simulink model "motor_modelo_prelab"  (R2017b)
settings: Solver=FixedStepAuto  StartTime=0.0  StopTime=150  FixedStep=1/fs  RelTol=1e-3
values from neighbouring files (symbols this model uses):
  den_c = denc    [lab3.m]
  den_filtro = den2    [lab3.m]
  den_motor = den1    [lab3.m]
  fs = 100    [lab3.m]    (also in script_motor.m = 10000; script_tanks.m = 1000)
  num_c = numc    [lab3.m]
  num_filtro = [1]    [lab3.m]
  num_motor = nump    (= 41.4)    [lab3.m]
settings Model: Creator=adgp97  LastModifiedBy=adgp97

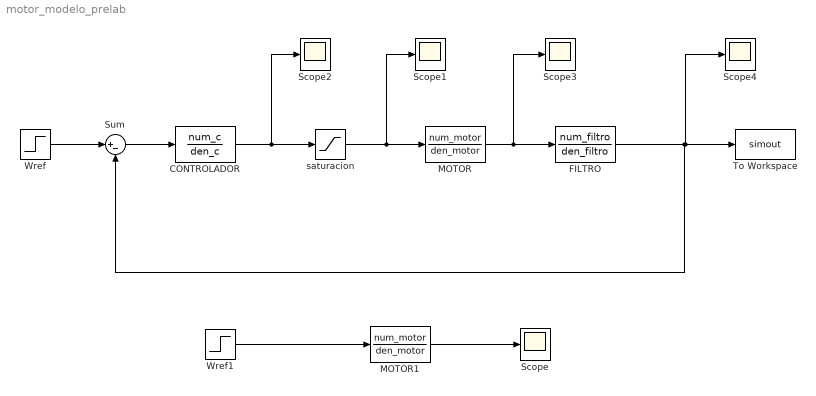
== system motor_modelo_prelab ==
  CONTROLADOR : TransferFcn  Numerator=num_c  Denominator=den_c
  FILTRO : TransferFcn  Numerator=num_filtro  Denominator=den_filtro
  MOTOR : TransferFcn  Numerator=num_motor  Denominator=den_motor
  MOTOR1 : TransferFcn  Numerator=num_motor  Denominator=den_motor
  Scope{,1..4} (5 alike) : Scope
  Sum : Sum  Inputs=|+-
  To Workspace : ToWorkspace  VariableName=simout  SampleTime=1/fs
      settings: Save2DSignal=2-D array (concatenate along first dimension)
  Wref : Step  Time=30  Before=102  After=112  SampleTime=1/fs
  Wref1 : Step  Time=30  Before=5.1  After=5.6  SampleTime=1/fs
  saturacion : Saturate  UpperLimit=10  LowerLimit=0
  wires:
  saturacion/1 -> Scope1/1, MOTOR/1
  MOTOR/1 -> Scope3/1, FILTRO/1
  Wref/1 -> Sum/1
  Sum/1 -> CONTROLADOR/1
  FILTRO/1 -> Sum/2, Scope4/1, To Workspace/1
  Wref1/1 -> MOTOR1/1
  MOTOR1/1 -> Scope/1
  CONTROLADOR/1 -> saturacion/1, Scope2/1
